simulink model "wrist_flexion"  (Simulink 6.6)
settings: Solver=ode3  SolverMode=SingleTasking  StartTime=0.0  StopTime=Inf  FixedStep=.001  RelTol=1e-3
libraries: xpclib x8, xpcnilib x4, simulink x4, limblab x3, dsparch4 x2
settings Model: Creator=Selket  LastModifiedBy=limblab  ExtModeArmWhenConnect=off  BufferReuse=off
settings OptimizationCC: BlockReduction=off  OptimizeBlockIOStorage=off  BufferReuse=off  ExpressionFolding=off  FoldNonRolledExpr=off  LocalBlockOutputs=off
settings DebuggingCC: MultiTaskCondExecSysMsg=none  StrictBusMsg=None
settings RTWCC: SystemTargetFile=xpctarget.tlc  TemplateMakefile=xpc_default_tmf  Description=xPC Target  ProcessScript=xpctarget_make_rtw_hook  IncludeERTFirstTime=on
settings xpcTargetCC: TargetFcnLib=ansi_tfl_tmw.mat  GenFloatMathFcnCalls=ANSI_C  PortableWordSizes=off  xPCisDownloadable=off  xPCisDefaultEnv=off

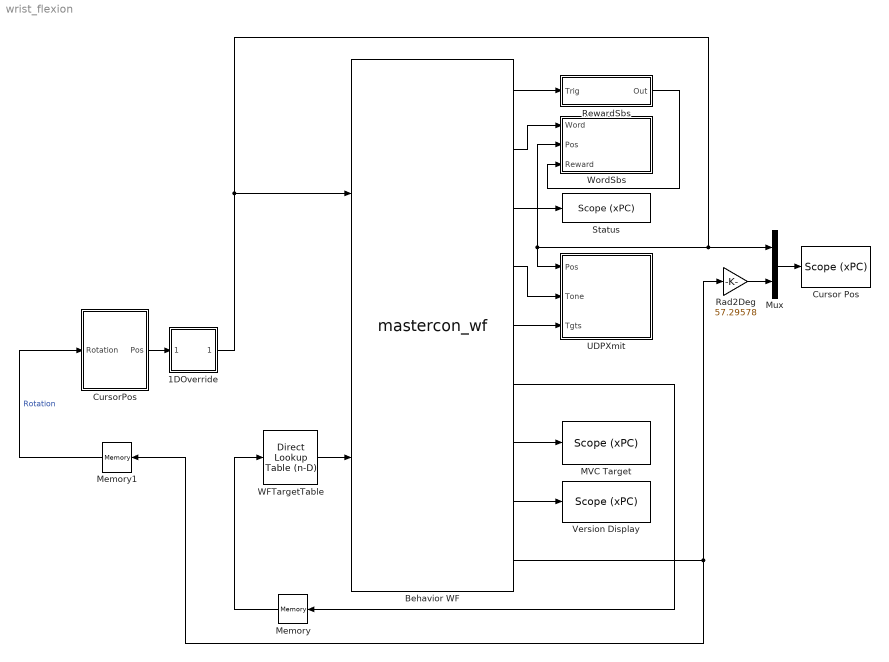
== system wrist_flexion ==
  1DOverride : Subsystem
  Behavior WF : S-Function  FunctionName=mastercon_wf  Parameters=8 5 .5 .5 1 2 2 2 2 2 0 0 0 0 0 0 0 0.7854 0
      mask Display:
      | disp('Master Control\nWrist-Flexion')
      | port_label('input',1,'cursor')
      | port_label('input',2,'target list')
      | port_label('output',1,'Reward')
      | port_label('output',2,'Word')
      | port_label('output',3,'Status')
      | port_label('output',4,'Tone')
      | port_label('output',5,'Targets')
      | port_label('output',6,'Target Select')
      | port_label('output',7,'MVC Target')
      | port_label('output',8,'version')
      | port_label('output',9,'rotation')
  Cursor Pos : xpclib/Misc./Scope (xPC)   SystemSampleTime=-1  scopeno=2  scopetype=Target  autostart=on  viewmode=Numerical  formatstr="' X: %4.6f   , Y: %4.6f   , (Rotated %6.2f degrees)  '"  grid=on  ylimits=[-10,10]  nosamples=10  noprepostsamples=0  interleave=10  triggermode=FreeRun  triggersignal=1  triggerlevel=0.0  triggerslope=Either  triggerscope=1  triggersample=0  filename=data.dat  mode=Lazy  writesize=512  autorestart=off
  CursorPos : Subsystem
  MVC Target : xpclib/Misc./Scope (xPC)   SystemSampleTime=-1  scopeno=6  scopetype=Target  autostart=on  viewmode=Numerical  formatstr="' Quad 1: %6.4f X  , Quad 1: %6.4f Y  , Quad 2: %6.4f X  , Quad 2: %6.4f Y  , Quad 3: %6.4f X  , Quad 3: %6.4f Y  , Quad 4: %6.4f X  , Quad 4: %6.4f Y  '"  grid=on  ylimits=[-10,10]  nosamples=10  noprepostsamples=0  interleave=10  triggermode=FreeRun  triggersignal=1  triggerlevel=0.0  triggerslope=Either  triggerscope=1  triggersample=0  filename=data.dat  mode=Lazy  writesize=512  autorestart=off
  Memory : Memory  Orientation=left  InheritSampleTime=on
  Memory1 : Memory  Orientation=left  InheritSampleTime=on
  Mux : Mux  Inputs=2
  Rad2Deg : Gain  Gain=57.29578
  RewardSbs : Subsystem
  Status : xpclib/Misc./Scope (xPC)   SystemSampleTime=-1  scopeno=1  scopetype=Target  autostart=on  viewmode=Numerical  formatstr='%6.0f State,%6.0f Rewards,%6.0f Aborts,%6.0f Failures'  grid=on  ylimits=[-10,10]  nosamples=10  noprepostsamples=0  interleave=10  triggermode=FreeRun  triggersignal=1  triggerlevel=0.0  triggerslope=Either  triggerscope=1  triggersample=0  filename=data.dat  mode=Lazy  writesize=512  autorestart=off
  UDPXmit : Subsystem
  Version Display : xpclib/Misc./Scope (xPC)   SystemSampleTime=-1  scopeno=4  scopetype=Target  autostart=on  viewmode=Numerical  formatstr='%6.0f major,%6.0f minor,%6.0f revision,%6.0f build'  grid=on  ylimits=[-10,10]  nosamples=10  noprepostsamples=0  interleave=10  triggermode=FreeRun  triggersignal=1  triggerlevel=0.0  triggerslope=Either  triggerscope=1  triggersample=0  filename=data.dat  mode=Lazy  writesize=512  autorestart=off
  WFTargetTable : simulink/Lookup Tables/Direct Lookup Table (n-D)  maskTabDims=2  explicitNumDims=1  outDims=Column  tabIsInput=off  mxTable=[5 5 5 5 5 5 5 5 5 5 5 5 5 5 5 5;5 5 5 5 5 5 5 5 5 5 5 5 5 5 5 5;5 5 5 5 5 5 5 5 5 5 5 5 5 5 5 5;5 5 5 5 5 5 5 5 5 5 5 5 5 5 5 5;0 0 0 0 0 0 0 0 0 0 0 0 0 0 0 0;0 0 0 0 0 0 0 0 0 0 0 0 0 0 0 0]  clipFlag=Warning  samptime=-1
  WordSbs : Subsystem
  wires:
  Behavior WF/2 -> WordSbs/1(Word)
  Behavior WF/1 -> RewardSbs/1(Trig)
  Memory/1 -> WFTargetTable/1
  WFTargetTable/1 -> Behavior WF/2
  Behavior WF/3 -> Status/1
  Behavior WF/4 -> UDPXmit/2(Tone)
  Behavior WF/5 -> UDPXmit/3(Tgts)
  CursorPos/1(Pos) -> 1DOverride/1(Trig)
  Behavior WF/6 -> Memory/1
  Behavior WF/7 -> MVC Target/1
  Behavior WF/8 -> Version Display/1
  1DOverride/1(Out1) -> Behavior WF/1, Mux/1, UDPXmit/1(Pos), WordSbs/2(Pos)
  Behavior WF/9 -> Memory1/1, Rad2Deg/1
  Memory1/1 -> CursorPos/1(Rotation)  "Rotation"
  Mux/1 -> Cursor Pos/1
  Rad2Deg/1 -> Mux/2
  RewardSbs/1(Out) -> WordSbs/3(Reward)

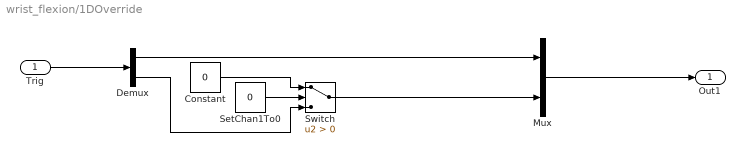
== system wrist_flexion/1DOverride ==
  Trig : Inport
  Constant : Constant  Value=0
  Demux : Demux  Outputs=2
  Mux : Mux  Inputs=2
  SetChan1To0 : Constant  Value=0
  Switch : Switch  Criteria=u2 > Threshold
  Out1 : Outport
  wires:
  Trig/1 -> Demux/1
  Switch/1 -> Mux/2
  Demux/1 -> Mux/1
  Mux/1 -> Out1/1
  SetChan1To0/1 -> Switch/2
  Constant/1 -> Switch/1
  Demux/2 -> Switch/3

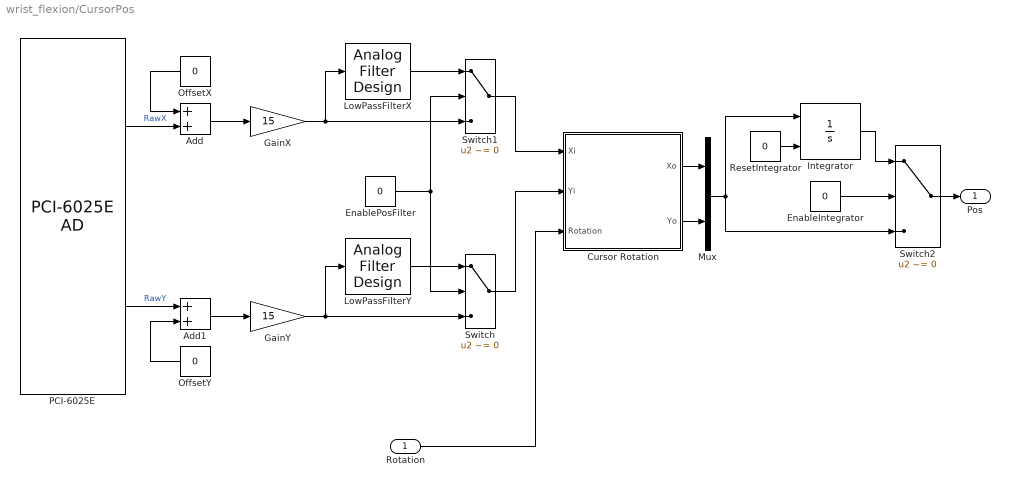
== system wrist_flexion/CursorPos ==
  Rotation : Inport
  Add : Sum  OutScaling=2^-10
  Add1 : Sum  OutScaling=2^-10
  Cursor Rotation : Subsystem
  EnableIntegrator : Constant  Value=0
  EnablePosFilter : Constant  Value=0
  GainX : Gain  Gain=15
  GainY : Gain  Gain=15
  Integrator : Integrator  ExternalReset=rising  LimitOutput=on  UpperSaturationLimit=15  LowerSaturationLimit=-15
  LowPassFilterX : dsparch4/Analog Filter Design  method=Butterworth  filttype=Lowpass  N=8  Wlo=30  Whi=80  Rp=2  Rs=40
  LowPassFilterY : dsparch4/Analog Filter Design  method=Butterworth  filttype=Lowpass  N=8  Wlo=30  Whi=80  Rp=2  Rs=40
  Mux : Mux  Inputs=2
  OffsetX : Constant  Orientation=left  Value=0
  OffsetY : Constant  Orientation=left  Value=0
  "PCI-6025E " : xpcnilib/A//D/PCI-6025E AD  channel=[9 10]  range=[-10]  coupling=[0]  sampletime=0.001  slot=-1
  ResetIntegrator : Constant  Value=0
  Switch : Switch  Criteria=u2 ~= 0
  Switch1 : Switch  Criteria=u2 ~= 0
  Switch2 : Switch  Criteria=u2 ~= 0
  Pos : Outport
  wires:
  "PCI-6025E "/1 -> Add/2  "RawX"
  "PCI-6025E "/2 -> Add1/1  "RawY"
  OffsetX/1 -> Add/1
  OffsetY/1 -> Add1/2
  Add/1 -> GainX/1
  LowPassFilterX/1 -> Switch1/1
  Add1/1 -> GainY/1
  LowPassFilterY/1 -> Switch/1
  EnablePosFilter/1 -> Switch/2, Switch1/2
  GainY/1 -> Switch/3, LowPassFilterY/1
  GainX/1 -> Switch1/3, LowPassFilterX/1
  Switch1/1 -> Cursor Rotation/1(Xi)
  Cursor Rotation/1(Xo) -> Mux/1
  Switch/1 -> Cursor Rotation/2(Yi)
  Cursor Rotation/2(Yo) -> Mux/2
  EnableIntegrator/1 -> Switch2/2
  Mux/1 -> Switch2/3, Integrator/1
  Switch2/1 -> Pos/1
  Integrator/1 -> Switch2/1
  ResetIntegrator/1 -> Integrator/2
  Rotation/1 -> Cursor Rotation/3(Rotation)

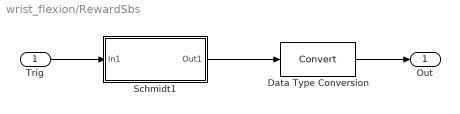
== system wrist_flexion/RewardSbs ==
  Trig : Inport
  Data Type Conversion : DataTypeConversion
  Schmidt1 : Subsystem  mask(Schmidt Trigger){Time=.3}
      mask help: Creates an output pulse of the specified time in seconds when trig goes high
      mask Help: Creates an output pulse of the specified time in seconds when trig goes high
      mask Display:
      | port_label('output',1,'out')
      | port_label('input',1,'trig')
      | fprintf('t = %.2f',Time)
  Out : Outport
  wires:
  Trig/1 -> Schmidt1/1(In1)
  Data Type Conversion/1 -> Out/1
  Schmidt1/1(Out1) -> Data Type Conversion/1

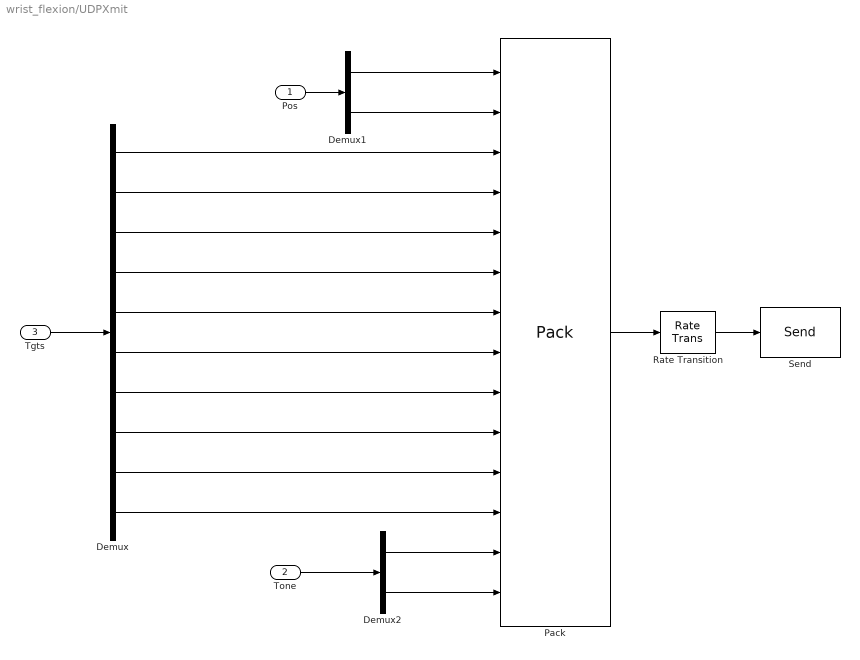
== system wrist_flexion/UDPXmit ==
  Pos : Inport
  Tone : Inport  Port=2
  Tgts : Inport  Port=3
  Demux : Demux  Outputs=10
  Demux1 : Demux  Outputs=2
  Demux2 : Demux  Outputs=2
  Pack : xpclib/UDP/Pack  datatypes={'double', 'double','double','double','double','double','double','double','double','double','double','double','double','double'}  byteAlign=1
  Rate Transition : RateTransition
  Send : xpclib/UDP/Send  ipAddress=192.168.0.2  ipPort=25000  localPort=-1  sampletime=.02
  wires:
  Rate Transition/1 -> Send/1
  Pack/1 -> Rate Transition/1
  Demux/10 -> Pack/12
  Demux/9 -> Pack/11
  Demux/8 -> Pack/10
  Demux/7 -> Pack/9
  Demux/6 -> Pack/8
  Demux/5 -> Pack/7
  Demux/4 -> Pack/6
  Demux/3 -> Pack/5
  Demux/2 -> Pack/4
  Demux/1 -> Pack/3
  Demux1/1 -> Pack/1
  Demux1/2 -> Pack/2
  Pos/1 -> Demux1/1
  Demux2/1 -> Pack/13
  Demux2/2 -> Pack/14
  Tone/1 -> Demux2/1
  Tgts/1 -> Demux/1

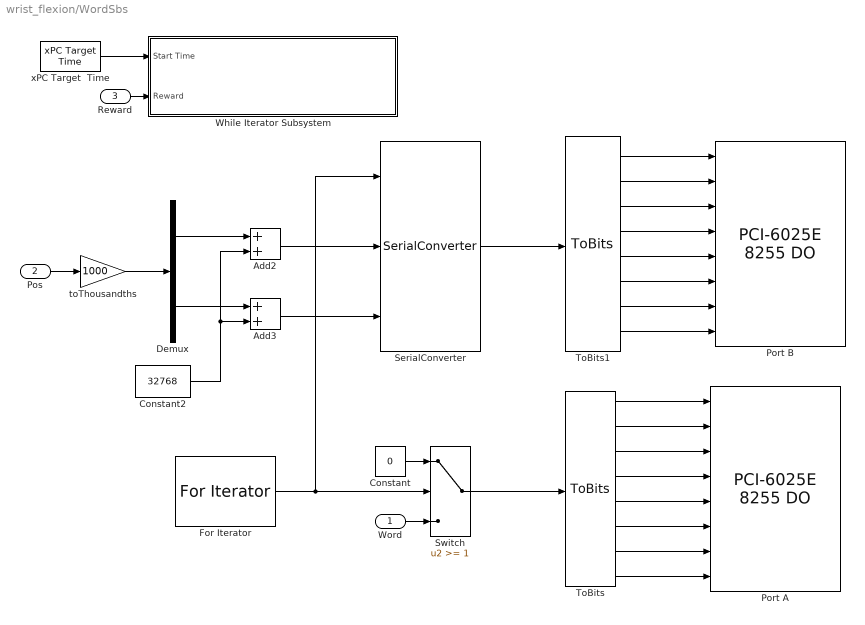
== system wrist_flexion/WordSbs ==
  Word : Inport
  Pos : Inport  Port=2
  Reward : Inport  Port=3
  Add2 : Sum  OutScaling=2^-10
  Add3 : Sum  OutScaling=2^-10
  Constant : Constant  Value=0
  Constant2 : Constant  Value=32768
  Demux : Demux  Outputs=2
  For Iterator : ForIterator  IterationLimit=4  IndexMode=Zero-based  IterationVariableDataType=double
  Port A : xpcnilib/Digital Output/PCI-6025E 8255 DO  channel=1:8  port=A  reset=[1]  initValue=[0]  chip=1  sampletime=-1  slot=[-1]
  Port B : xpcnilib/Digital Output/PCI-6025E 8255 DO  channel=1:8  port=B  reset=[1]  initValue=[0]  chip=1  sampletime=-1  slot=-1
  SerialConverter : limblab/SerialConverter
  Switch : Switch  Threshold=1  ZeroCross=off
  ToBits : limblab/ToBits
  ToBits1 : limblab/ToBits
  While Iterator Subsystem : Subsystem  TreatAsAtomicUnit=on
  toThousandths : Gain  Gain=1000
  "xPC Target  Time " : xpclib/Misc./xPC Target  Time   ts=-1
  wires:
  ToBits/1 -> Port A/1
  ToBits/2 -> Port A/2
  ToBits/3 -> Port A/3
  ToBits/4 -> Port A/4
  ToBits/5 -> Port A/5
  ToBits/6 -> Port A/6
  ToBits/7 -> Port A/7
  ToBits/8 -> Port A/8
  Switch/1 -> ToBits/1
  For Iterator/1 -> Switch/2, SerialConverter/1
  "xPC Target  Time "/1 -> While Iterator Subsystem/1(Start Time)
  Constant/1 -> Switch/1
  Constant2/1 -> Add2/2, Add3/2
  ToBits1/8 -> Port B/8
  ToBits1/7 -> Port B/7
  ToBits1/6 -> Port B/6
  ToBits1/5 -> Port B/5
  ToBits1/1 -> Port B/1
  ToBits1/2 -> Port B/2
  ToBits1/3 -> Port B/3
  ToBits1/4 -> Port B/4
  SerialConverter/1 -> ToBits1/1
  Word/1 -> Switch/3
  Add2/1 -> SerialConverter/2
  Add3/1 -> SerialConverter/3
  Pos/1 -> toThousandths/1
  Demux/1 -> Add2/1
  Demux/2 -> Add3/1
  toThousandths/1 -> Demux/1
  Reward/1 -> While Iterator Subsystem/2(Reward)

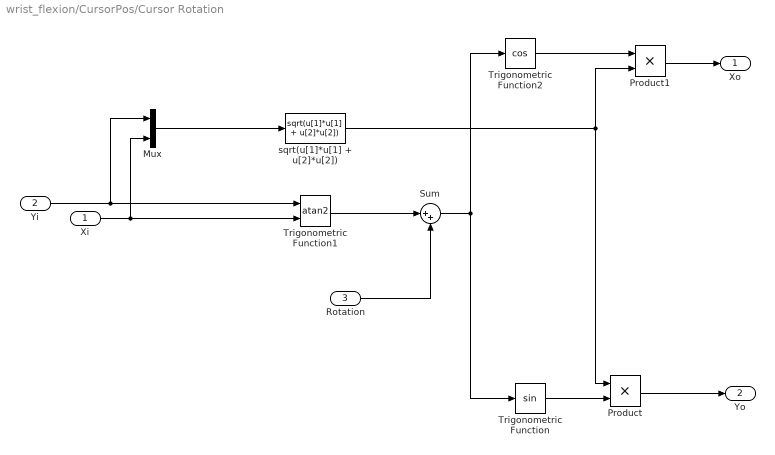
== system wrist_flexion/CursorPos/Cursor Rotation ==
  Xi : Inport
  Yi : Inport  Port=2
  Rotation : Inport  Port=3
  Mux : Mux  Inputs=2
  Product : Product  RndMeth=Zero
  Product1 : Product  RndMeth=Zero
  Sum : Sum  Inputs=|++
  Trigonometric Function : Trigonometry
  Trigonometric Function1 : Trigonometry  Operator=atan2
  Trigonometric Function2 : Trigonometry  Operator=cos
  sqrt(u[1]*u[1] + u[2]*u[2]) : Fcn  Expr=sqrt(u[1]*u[1] + u[2]*u[2])
  Xo : Outport
  Yo : Outport  Port=2
  wires:
  Rotation/1 -> Sum/2
  Trigonometric Function1/1 -> Sum/1
  Yi/1 -> Trigonometric Function1/1, Mux/1
  Xi/1 -> Trigonometric Function1/2, Mux/2
  Mux/1 -> sqrt(u[1]*u[1] + u[2]*u[2])/1
  Trigonometric Function/1 -> Product/2
  Product/1 -> Yo/1
  sqrt(u[1]*u[1] + u[2]*u[2])/1 -> Product/1, Product1/2
  Sum/1 -> Trigonometric Function/1, Trigonometric Function2/1
  Product1/1 -> Xo/1
  Trigonometric Function2/1 -> Product1/1

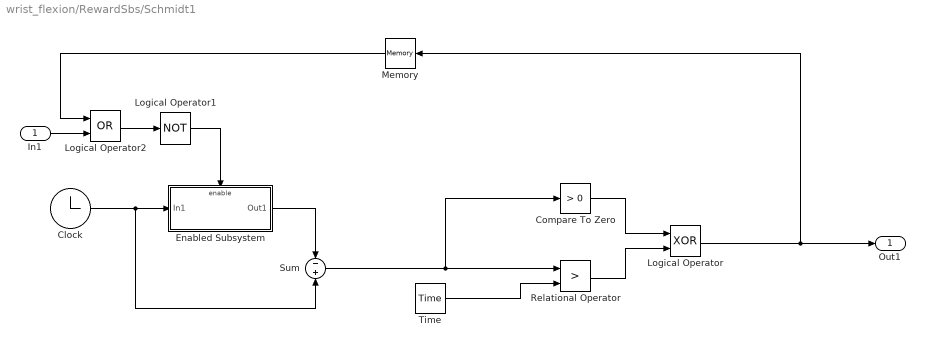
== system wrist_flexion/RewardSbs/Schmidt1 ==
  In1 : Inport
  Clock : Clock
  Compare To Zero : simulink/Logic and Bit Operations/Compare To Zero  SystemSampleTime=-1  relop=>  LogicOutDataTypeMode=uint8  ZeroCross=off
  Enabled Subsystem : Subsystem  TreatAsAtomicUnit=on
  Logical Operator : Logic  Operator=XOR  AllPortsSameDT=off  OutDataTypeMode=Boolean  SampleTime=.001
  Logical Operator1 : Logic  Operator=NOT  AllPortsSameDT=off  OutDataTypeMode=Boolean
  Logical Operator2 : Logic  Operator=OR  AllPortsSameDT=off  OutDataTypeMode=Boolean  SampleTime=.001
  Memory : Memory  Orientation=left
  Relational Operator : RelationalOperator  Operator=>  LogicOutDataTypeMode=Boolean
  Sum : Sum  Inputs=-+
  Time : Constant  Value=Time
  Out1 : Outport
  wires:
  Clock/1 -> Enabled Subsystem/1(In1), Sum/2
  Enabled Subsystem/1(Out1) -> Sum/1
  Sum/1 -> Compare To Zero/1, Relational Operator/1
  Time/1 -> Relational Operator/2
  Compare To Zero/1 -> Logical Operator/1
  Relational Operator/1 -> Logical Operator/2
  Logical Operator1/1 -> Enabled Subsystem/Enable
  Logical Operator/1 -> Out1/1, Memory/1
  In1/1 -> Logical Operator2/2
  Logical Operator2/1 -> Logical Operator1/1
  Memory/1 -> Logical Operator2/1

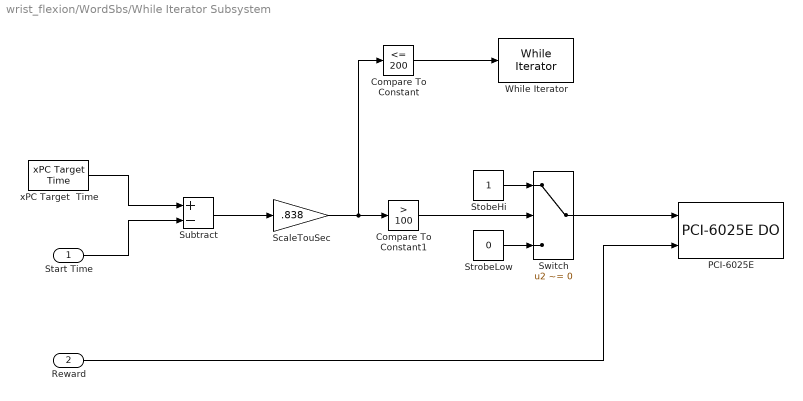
== system wrist_flexion/WordSbs/While Iterator Subsystem ==
  Start Time : Inport
  Reward : Inport  Port=2
  Compare To Constant : simulink/Logic and Bit Operations/Compare To Constant  SystemSampleTime=-1  relop=<=  const=200  LogicOutDataTypeMode=boolean
  Compare To Constant1 : simulink/Logic and Bit Operations/Compare To Constant  SystemSampleTime=-1  relop=>  const=100  LogicOutDataTypeMode=boolean  ZeroCross=off
  "PCI-6025E " : xpcnilib/Digital Output/PCI-6025E DO  channel=[1 2]  reset=[1]  initValue=[0]  sampletime=-1  slot=-1
  ScaleTouSec : Gain  Gain=.838
  StobeHi : Constant
  StrobeLow : Constant  Value=0
  Subtract : Sum  Inputs=+-  OutScaling=2^-10
  Switch : Switch  Criteria=u2 ~= 0
  While Iterator : WhileIterator  MaxIters=-1  WhileBlockType=do-while
  "xPC Target  Time " : xpclib/Misc./xPC Target  Time   ts=-1
  wires:
  "xPC Target  Time "/1 -> Subtract/1
  Start Time/1 -> Subtract/2
  Subtract/1 -> ScaleTouSec/1
  Compare To Constant/1 -> While Iterator/1
  ScaleTouSec/1 -> Compare To Constant/1, Compare To Constant1/1
  Compare To Constant1/1 -> Switch/2
  StobeHi/1 -> Switch/1
  StrobeLow/1 -> Switch/3
  Switch/1 -> "PCI-6025E "/1
  Reward/1 -> "PCI-6025E "/2

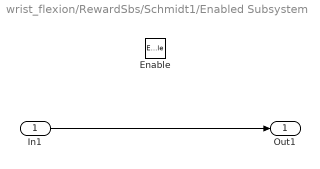
== system wrist_flexion/RewardSbs/Schmidt1/Enabled Subsystem ==
  In1 : Inport
  Enable : EnablePort
  Out1 : Outport
  wires:
  In1/1 -> Out1/1
